simulink model "model2021"  (R2021b)
settings: Solver=VariableStepAuto  StartTime=0.0  StopTime=10.0  RelTol=1e-3
values from neighbouring files (symbols this model uses):
  b = 0.11    [quadraptorModel.m]
  g = 9.80665    [quadraptorModel.m]
  I = diag([Ixx, Iyy, Izz])    [quadraptorModel.m]
  k = 2.165856918e-8    (= 2.165856918e-08)    [quadraptorModel.m]
  L = 0.0475    [quadraptorModel.m]
  m = drone_mass + optitrack_frame_mass    (= 0.067)    [quadraptorModel.m]
undefined symbols (not defined in the file or in its folder): Fd
libraries: matrix_library x1
settings Model: Creator=enriq  LastModifiedBy=enriq
settings DebuggingCC: UnconnectedInputMsg=none  UnconnectedOutputMsg=none  UnconnectedLineMsg=none
settings ModelReferenceCC: EnableRefExpFcnMdlSchedulingChecks=off
settings RTWCC: DLArmComputeVersion=20.02.1

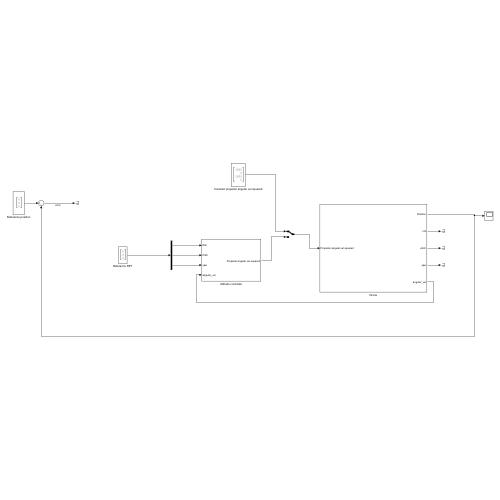
[thumbnail: Simulink's stored preview of the top-level diagram]
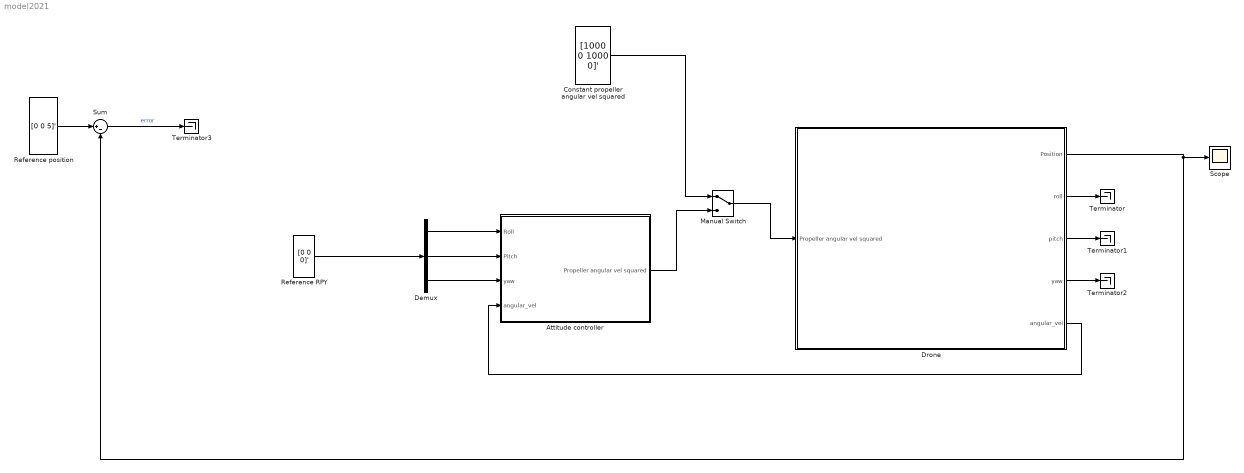
== system model2021 ==
  Attitude controller : Subsystem
  Constant propeller angular vel squared : Constant  Value=[1000 0 1000 0]'  VectorParams1D=off
  Demux : Demux  Outputs=3
  Drone : Subsystem
  Manual Switch : ManualSwitch
  Reference RPY : Constant  Value=[0 0 0]'  VectorParams1D=off
  Reference position : Constant  Value=[0 0 5]'  VectorParams1D=off
  Scope : Scope
  Sum : Sum  Inputs=|+-
  Terminator{,1..3} (4 alike) : Terminator
  wires:
  Drone/1(Position) -> Scope/1, Sum/2
  Drone/2(roll) -> Terminator/1
  Drone/3(pitch) -> Terminator1/1
  Drone/4(yaw) -> Terminator2/1
  Reference position/1 -> Sum/1
  Sum/1 -> Terminator3/1  "error"
  Constant propeller angular vel squared/1 -> Manual Switch/1
  Manual Switch/1 -> Drone/1(Propeller angular vel squared)
  Attitude controller/1(Propeller angular vel squared) -> Manual Switch/2
  Drone/5(angular_vel) -> Attitude controller/4(angular_vel)
  Demux/1 -> Attitude controller/1(Roll)
  Demux/2 -> Attitude controller/2(Pitch)
  Demux/3 -> Attitude controller/3(yaw)
  Reference RPY/1 -> Demux/1

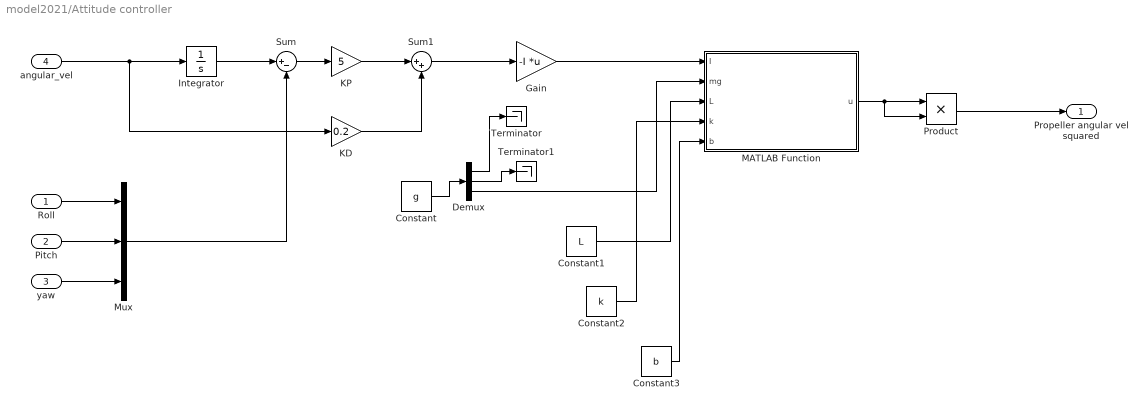
== system model2021/Attitude controller ==
  Roll : Inport
  Pitch : Inport  Port=2
  yaw : Inport  Port=3
  angular_vel : Inport  Port=4
  Constant : Constant  Value=g
  Constant1 : Constant  Value=L
  Constant2 : Constant  Value=k
  Constant3 : Constant  Value=b
  Demux : Demux  Outputs=3
  Gain : Gain  Gain=-I  Multiplication=Matrix(K*u)
  Integrator : Integrator
  KD : Gain  Gain=0.2
  KP : Gain  Gain=5
  MATLAB Function : MATLAB Function  TreatAsAtomicUnit=on
  Mux : Mux  Inputs=3
  Product : Product
  Sum : Sum  Inputs=|+-
  Sum1 : Sum  Inputs=|++
  Terminator : Terminator
  Terminator1 : Terminator
  Propeller angular vel squared : Outport
  wires:
  angular_vel/1 -> KD/1, Integrator/1
  Roll/1 -> Mux/1
  Pitch/1 -> Mux/2
  yaw/1 -> Mux/3
  Integrator/1 -> Sum/1
  Mux/1 -> Sum/2
  Sum/1 -> KP/1
  KP/1 -> Sum1/1
  KD/1 -> Sum1/2
  Sum1/1 -> Gain/1
  Constant/1 -> Demux/1
  Demux/3 -> MATLAB Function/2(mg)
  Gain/1 -> MATLAB Function/1(I)
  Demux/1 -> Terminator/1
  Demux/2 -> Terminator1/1
  Constant1/1 -> MATLAB Function/3(L)
  Constant2/1 -> MATLAB Function/4(k)
  Constant3/1 -> MATLAB Function/5(b)
  MATLAB Function/1(u) -> Product/2, Product/1
  Product/1 -> Propeller angular vel squared/1

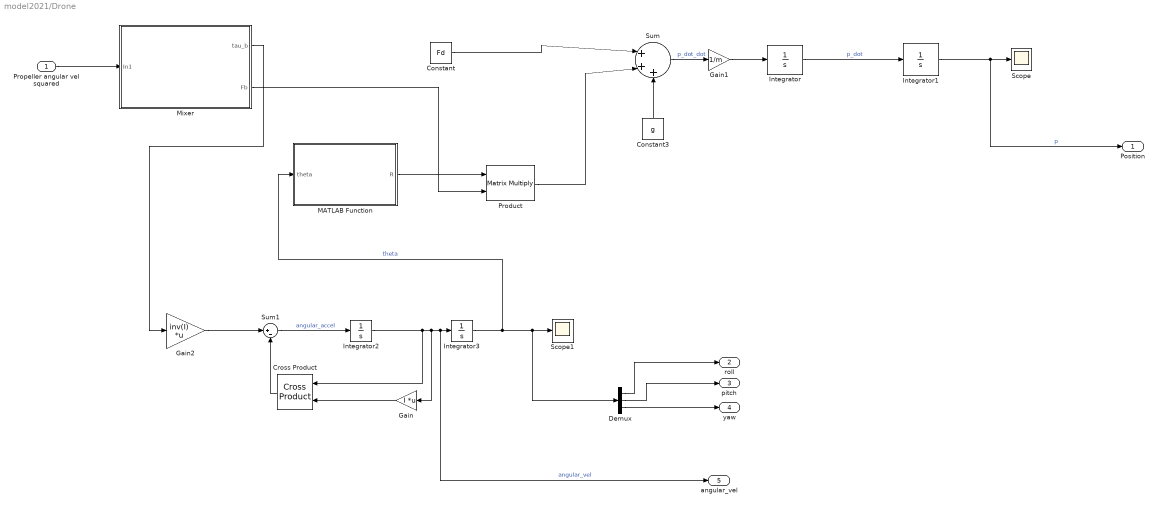
== system model2021/Drone ==
  Propeller angular vel squared : Inport
  Constant : Constant  Value=Fd
  Constant3 : Constant  Value=g
  Cross Product : matrix_library/Cross Product
  Demux : Demux  Outputs=3
  Gain : Gain  Gain=I  Multiplication=Matrix(K*u)
  Gain1 : Gain  Gain=1/m
  Gain2 : Gain  Gain=inv(I)  Multiplication=Matrix(K*u)
  Integrator{,1..3} (4 alike) : Integrator
  MATLAB Function : MATLAB Function  TreatAsAtomicUnit=on
  Mixer : Subsystem
  Product : Product  Multiplication=Matrix(*)
  Scope : Scope
  Scope1 : Scope
  Sum : Sum  Inputs=|+++
  Sum1 : Sum  Inputs=|+-
  Position : Outport
  roll : Outport  Port=2
  pitch : Outport  Port=3
  yaw : Outport  Port=4
  angular_vel : Outport  Port=5
  wires:
  Integrator2/1 -> Cross Product/1, angular_vel/1, Integrator3/1, Gain/1  "angular_vel"
  Sum1/1 -> Integrator2/1  "angular_accel"
  Gain2/1 -> Sum1/1
  Integrator1/1 -> Position/1, Scope/1  "p"
  Cross Product/1 -> Sum1/2
  Integrator/1 -> Integrator1/1  "p_dot"
  Gain/1 -> Cross Product/2
  Integrator3/1 -> MATLAB Function/1(theta), Demux/1, Scope1/1  "theta"
  Sum/1 -> Gain1/1  "p_dot_dot"
  Gain1/1 -> Integrator/1
  Constant3/1 -> Sum/3
  Demux/1 -> roll/1
  Demux/2 -> pitch/1
  Demux/3 -> yaw/1
  Propeller angular vel squared/1 -> Mixer/1(In1)
  MATLAB Function/1(R) -> Product/1
  Mixer/2(Fb) -> Product/2
  Product/1 -> Sum/2
  Mixer/1(tau_b) -> Gain2/1
  Constant/1 -> Sum/1

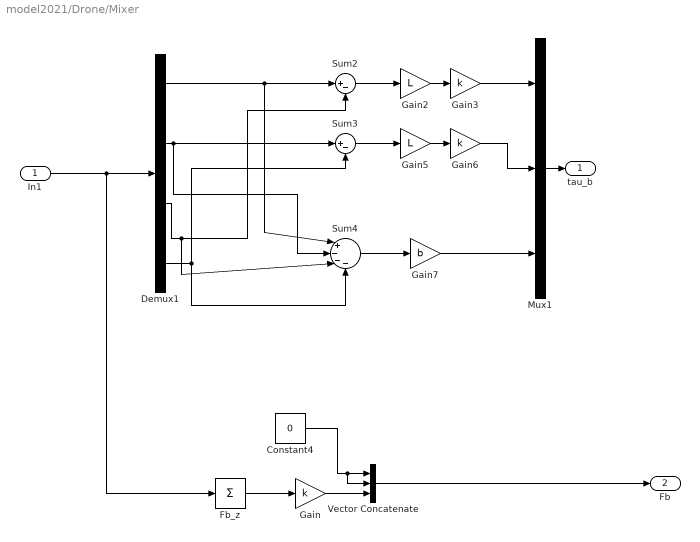
== system model2021/Drone/Mixer ==
  In1 : Inport
  Constant4 : Constant  Value=0
  Demux1 : Demux
  Fb_z : Sum  Inputs=+
  Gain : Gain  Gain=k
  Gain2 : Gain  Gain=L
  Gain3 : Gain  Gain=k
  Gain5 : Gain  Gain=L
  Gain6 : Gain  Gain=k
  Gain7 : Gain  Gain=b
  Mux1 : Mux  Inputs=3
  Sum2 : Sum  Inputs=|+-
  Sum3 : Sum  Inputs=|+-
  Sum4 : Sum  Inputs=|+---
  Vector Concatenate : Concatenate  NumInputs=3
  tau_b : Outport
  Fb : Outport  Port=2
  wires:
  Sum4/1 -> Gain7/1
  Demux1/2 -> Sum3/1, Sum4/2
  Sum2/1 -> Gain2/1
  Mux1/1 -> tau_b/1
  Demux1/3 -> Sum4/3, Sum2/2
  Demux1/1 -> Sum2/1, Sum4/1
  Demux1/4 -> Sum4/4, Sum3/2
  Sum3/1 -> Gain5/1
  Gain2/1 -> Gain3/1
  Gain5/1 -> Gain6/1
  Gain3/1 -> Mux1/1
  Gain7/1 -> Mux1/3
  Gain6/1 -> Mux1/2
  Constant4/1 -> Vector Concatenate/2, Vector Concatenate/1
  Fb_z/1 -> Gain/1
  In1/1 -> Fb_z/1, Demux1/1
  Vector Concatenate/1 -> Fb/1
  Gain/1 -> Vector Concatenate/3

== matlab function model2021/Attitude controller/MATLAB Function ==
  data: I input; u output; mg input; L input; k input; b input
function u = computeControlAction(I, mg, L, k, b)

I = [I; mg/k];

A = [L*k,  0,  -L*k,   0;
     0,   L*k,  0,   -L*k;
     b,   -b,   b,     -b;
     1,    1,   1,      1];

u = A\I;

== matlab function model2021/Drone/MATLAB Function ==
  data: theta input; R output
function R = computeRotationMatrix(theta)

Rx = [1     0               0;
      0 cos(theta(1)) -sin(theta(1));
      0 sin(theta(1))  cos(theta(1))];

Ry = [cos(theta(2))     0         sin(theta(2));
      0                 1               0;
      -sin(theta(2))    0         cos(theta(1))];

Rz = [cos(theta(1)) -sin(theta(1))    0;
      sin(theta(1))  cos(theta(1))    0;
          0               0           1];


R = Rx * Ry * Rz;
